simulink model "siso_4_channel_teleop_force"  (R2021a)
settings: Solver=VariableStepAuto  StartTime=0.0  StopTime=5  FixedStep=Ts  RelTol=1e-3
values from neighbouring files (symbols this model uses):
  A = pi/4    (= 0.785398163397)    [assignment2.m]
  Be = 100    [assignment2.m]
  Bh = 7    [assignment2.m]
  Bm = 100    [assignment2.m]
  Bs = 1000    [assignment2.m]
  Cmf = -0.67    [assignment2.m]
  Csf = -0.67    [assignment2.m]
  Dh = 500    [assignment2.m]
  Dm = 0    [assignment2.m]
  Ds = 0    [assignment2.m]
  Fc = 1    [assignment2.m]
  Flp = 5    [assignment2.m]
  Jh = 0.05    [assignment2.m]
  k_h = 8000    [assignment2.m]
  Ke = 200    [assignment2.m]
  Kh = 200    [assignment2.m]
  Km = 500    [assignment2.m]
  Ks = 80000    [assignment2.m]
  Mm = 0.5    [assignment2.m]
  Ms = 2    [assignment2.m]
  Ts = 0.001    [assignment2.m]
  xe = 1    [assignment2.m]
libraries: simulink x2
settings Model: Creator=fabio  LastModifiedBy=fabio

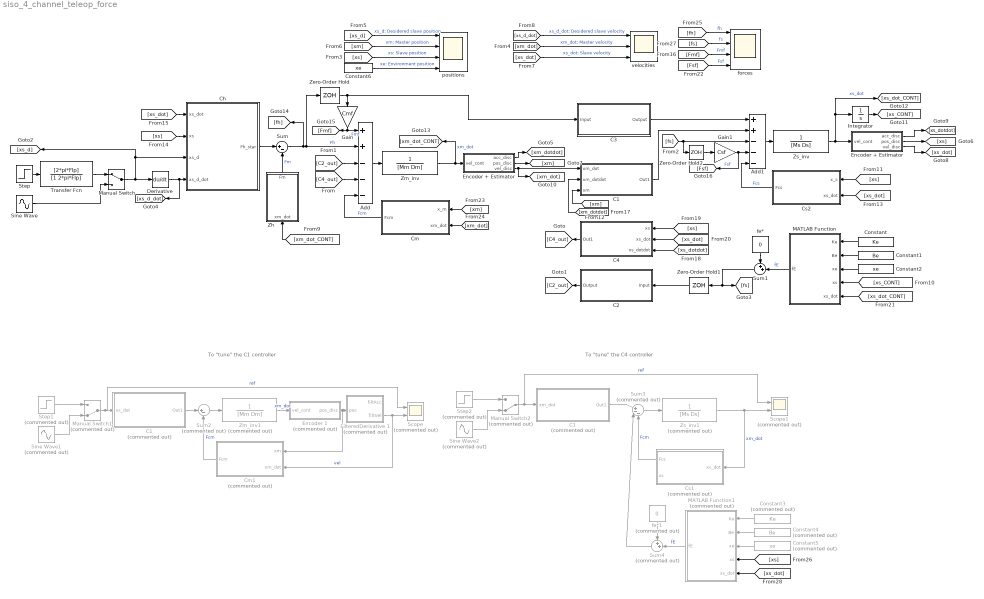
== system siso_4_channel_teleop_force ==
  note: To "tune" the C1 controller
  note: To "tune" the C4 controller
  Add : Sum  Inputs=++---
  Add1 : Sum  Inputs=++---
  C1 : Subsystem
  "C1 " : Subsystem  Commented=on
  "C1    " : Subsystem  Commented=on
  C2 : Subsystem
  C3 : Subsystem
  C4 : Subsystem
  Ch : Subsystem
  Cm : Subsystem
  Cm1 : Subsystem  Commented=on
  Constant : Constant  Value=Ke
  Constant1 : Constant  Value=Be
  Constant2 : Constant  Value=xe
  Constant3 : Constant  Commented=on  Value=Ke
  Constant4 : Constant  Commented=on  Value=Be
  Constant5 : Constant  Commented=on  Value=xe
  Constant6 : Constant  Value=xe
  Cs1 : Subsystem  Commented=on
  Cs2 : Subsystem
  Derivative : Derivative
  Encoder + Estimator : Subsystem
  "Encoder + Estimator " : Subsystem
  Encoder 1 : Subsystem  Commented=on
  FilteredDerivative 1 : Subsystem  Commented=on
  Gain : Gain  Gain=Cmf
  Gain1 : Gain  Gain=Csf
  Integrator : Integrator
  MATLAB Function : MATLAB Function  TreatAsAtomicUnit=on
  MATLAB Function1 : MATLAB Function  Commented=on  TreatAsAtomicUnit=on
  Manual Switch : ManualSwitch
  Manual Switch1 : ManualSwitch  Commented=on  CurrentSetting=0
  Manual Switch2 : ManualSwitch  Commented=on  CurrentSetting=0
  Scope : Scope  Commented=on  NumInputPorts=2
  Scope1 : Scope  Commented=on  NumInputPorts=2
  Sine Wave : Sin  Amplitude=A  Frequency=Fc*2*pi  SampleTime=0
  Sine Wave1 : Sin  Commented=on  Amplitude=A  Frequency=Fc  SampleTime=0
  Sine Wave2 : Sin  Commented=on  Amplitude=A  Frequency=Fc  SampleTime=0
  Step : Step  After=A  SampleTime=0
  Step1 : Step  Commented=on  SampleTime=0
  Step2 : Step  Commented=on  SampleTime=0
  Sum : Sum  Inputs=|+-
  Sum1 : Sum  Inputs=++|
  Sum2 : Sum  Commented=on  Inputs=|+-
  Sum3 : Sum  Commented=on  Inputs=|+--
  Sum4 : Sum  Commented=on  Inputs=++|
  Transfer Fcn : TransferFcn  Numerator=[2*pi*Flp]  Denominator=[1 2*pi*Flp]
  Zero-Order Hold : ZeroOrderHold  SampleTime=Ts
  Zero-Order Hold1 : ZeroOrderHold  SampleTime=Ts
  Zero-Order Hold2 : ZeroOrderHold  SampleTime=Ts
  Zh : Subsystem
  Zm_inv : TransferFcn  Numerator=[0 1]  Denominator=[Mm Dm]
  Zm_inv1 : TransferFcn  Commented=on  Numerator=[0 1]  Denominator=[Mm Dm]
  Zs_inv : TransferFcn  Numerator=[0 1]  Denominator=[Ms Ds]
  Zs_inv1 : TransferFcn  Commented=on  Numerator=[0 1]  Denominator=[Ms Ds]
  fe* : Constant  Value=0
  fe*1 : Constant  Commented=on  Value=0
  forces : Scope  NumInputPorts=4
  positions : Scope  NumInputPorts=4
  velocities : Scope  NumInputPorts=3
  wires:
  Zh/1(Fm) -> Sum/2  "Fm"
  Sum/1 -> Add/2, Zero-Order Hold/1, [fh]  "Fh"
  Add/1 -> Zm_inv/1
  Cm/1(Fcm) -> Add/5  "Fcm"
  Cs2/1(Fcs) -> Add1/5  "Fcs"
  Add1/1 -> Zs_inv/1
  Constant/1 -> MATLAB Function/1(Ke)
  Constant1/1 -> MATLAB Function/2(Be)
  Constant2/1 -> MATLAB Function/3(xe)
  [xs_CONT] -> MATLAB Function/4(xs)
  [xs_dot_CONT] -> MATLAB Function/5(xs_dot)
  MATLAB Function/1(fE) -> Sum1/2  "fE"
  C4/1(Out1) -> [C4_out]
  [C4_out] -> Add/4
  C3/1(Output) -> Add1/1
  [fs] -> Add1/3, Zero-Order Hold2/1
  C2/1(Output) -> [C2_out]
  Ch/1(Fh_star) -> Sum/1
  [C2_out] -> Add/3
  [xs_d] -> positions/1  "xs_d: Desidered slave position"
  [xm] -> positions/2  "xm: Master position"
  [xs] -> positions/3  "xs: Slave position"
  [xm_dot] -> velocities/2  "xm_dot: Master velocity"
  [xs_dot] -> velocities/3  "xs_dot: Slave velocity"
  [xs_d_dot] -> velocities/1  "xs_d_dot: Desidered slave velocity"
  [xs_dot] -> Ch/4(xs_dot)
  [xs] -> Ch/3(xs)
  Sine Wave/1 -> Manual Switch/2
  Derivative/1 -> [xs_d_dot], Ch/1(xs_d_dot)
  fe*/1 -> Sum1/1
  Sum2/1 -> Zm_inv1/1
  Cm1/1(Fcm) -> Sum2/2  "Fcm"
  "C1    "/1(Out1) -> Sum2/1
  Step1/1 -> Manual Switch1/1
  Sine Wave1/1 -> Manual Switch1/2
  Manual Switch1/1 -> Scope/1, "C1    "/1(xs_dot)  "ref"
  Manual Switch2/1 -> "C1 "/1(xm_dot), Scope1/1  "ref"
  Sine Wave2/1 -> Manual Switch2/2
  Step2/1 -> Manual Switch2/1
  "C1 "/1(Out1) -> Sum3/1
  Zs_inv1/1 -> Cs1/1(xs_dot), Scope1/2  "xm_dot"
  Sum3/1 -> Zs_inv1/1
  fe*1/1 -> Sum4/1
  [xs] -> MATLAB Function1/4(xs)
  MATLAB Function1/1(fE) -> Sum4/2  "fE"
  Constant3/1 -> MATLAB Function1/1(Ke)
  [xs_dot] -> MATLAB Function1/5(xs_dot)
  Constant4/1 -> MATLAB Function1/2(Be)
  Constant5/1 -> MATLAB Function1/3(xe)
  Cs1/1(Fcs) -> Sum3/3  "Fcm"
  Sum4/1 -> Sum3/2
  Step/1 -> Transfer Fcn/1
  Transfer Fcn/1 -> Manual Switch/1
  Zs_inv/1 -> [xs_dot_CONT], Integrator/1, "Encoder + Estimator "/1(vel_cont)  "xs_dot"
  Zm_inv/1 -> [xm_dot_CONT], Encoder + Estimator/1(vel_cont)  "xm_dot"
  "Encoder + Estimator "/3(vel_disc) -> [xs_dot]
  Zero-Order Hold1/1 -> C2/1(Input)
  Manual Switch/1 -> Ch/2(xs_d), [xs_d], Derivative/1
  "Encoder + Estimator "/1(acc_disc) -> [xs_dotdot]
  [xs] -> C4/1(xs)
  [xs_dotdot] -> C4/3(xs_dotdot)
  [xs_dot] -> C4/2(xs_dot)
  Integrator/1 -> [xs_CONT]
  [xs] -> Cs2/1(x_s)
  [xs_dot] -> Cs2/2(xs_dot)
  Zero-Order Hold/1 -> Gain/1, C3/1(Input)
  Encoder + Estimator/1(acc_disc) -> [xm_dotdot]
  [xm] -> C1/3(xm)
  [xm_dotdot] -> C1/2(xm_dotdot)
  Sum1/1 -> [fs], Zero-Order Hold1/1
  [xm] -> Cm/1(x_m)
  [xm_dot] -> Cm/2(xm_dot)
  Zm_inv1/1 -> Encoder 1/1(vel_cont)  "xm_dot"
  Encoder 1/1(pos_disc) -> Cm1/1(xm), FilteredDerivative 1/1(pos)
  FilteredDerivative 1/2(filtVel) -> Cm1/2(xm_dot), Scope/2  "vel"
  [xm_dot_CONT] -> Zh/1(xm_dot)
  C1/1(Out1) -> Add1/2
  Encoder + Estimator/3(vel_disc) -> C1/1(xm_dot), [xm_dot]
  Encoder + Estimator/2(pos_disc) -> [xm]
  "Encoder + Estimator "/2(pos_disc) -> [xs]
  Constant6/1 -> positions/4  "xe: Environment position"
  [fh] -> forces/1  "fh"
  [fs] -> forces/2  "fs"
  Gain/1 -> Add/1, [Fmf]  "Fmf"
  Gain1/1 -> [Fsf], Add1/4  "Fsf"
  Zero-Order Hold2/1 -> Gain1/1
  [Fmf] -> forces/3  "Fmf"
  [Fsf] -> forces/4  "Fsf"

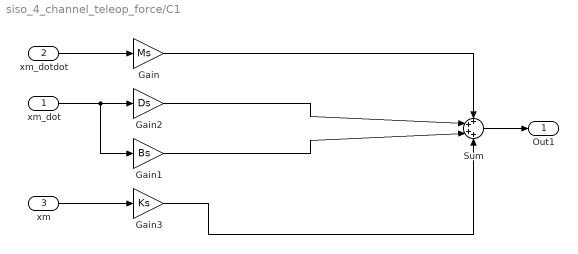
== system siso_4_channel_teleop_force/C1 ==
  xm_dot : Inport
  xm_dotdot : Inport  Port=2
  xm : Inport  Port=3
  Gain : Gain  Gain=Ms
  Gain1 : Gain  Gain=Bs
  Gain2 : Gain  Gain=Ds
  Gain3 : Gain  Gain=Ks
  Sum : Sum  Inputs=++++
  Out1 : Outport
  wires:
  Gain/1 -> Sum/1
  Gain2/1 -> Sum/2
  Gain1/1 -> Sum/3
  Gain3/1 -> Sum/4
  Sum/1 -> Out1/1
  xm/1 -> Gain3/1
  xm_dot/1 -> Gain1/1, Gain2/1
  xm_dotdot/1 -> Gain/1

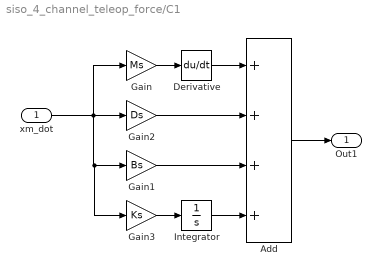
== system siso_4_channel_teleop_force/C1  ==
  xm_dot : Inport
  Add : Sum  Inputs=++++
  Derivative : Derivative
  Gain : Gain  Gain=Ms
  Gain1 : Gain  Gain=Bs
  Gain2 : Gain  Gain=Ds
  Gain3 : Gain  Gain=Ks
  Integrator : Integrator
  Out1 : Outport
  wires:
  Add/1 -> Out1/1
  Integrator/1 -> Add/4
  Gain3/1 -> Integrator/1
  Gain1/1 -> Add/3
  Gain2/1 -> Add/2
  Derivative/1 -> Add/1
  Gain/1 -> Derivative/1
  xm_dot/1 -> Gain2/1, Gain1/1, Gain3/1, Gain/1

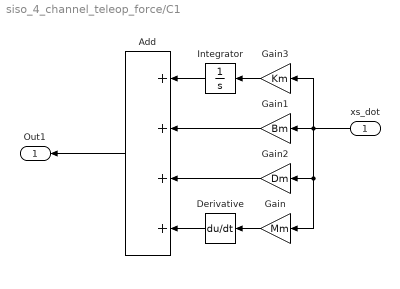
== system siso_4_channel_teleop_force/C1     ==
  xs_dot : Inport
  Add : Sum  Inputs=++++
  Derivative : Derivative
  Gain : Gain  Gain=Mm
  Gain1 : Gain  Gain=Bm
  Gain2 : Gain  Gain=Dm
  Gain3 : Gain  Gain=Km
  Integrator : Integrator
  Out1 : Outport
  wires:
  Add/1 -> Out1/1
  Integrator/1 -> Add/1
  Gain1/1 -> Add/2
  Gain2/1 -> Add/3
  Derivative/1 -> Add/4
  xs_dot/1 -> Gain1/1, Gain3/1, Gain2/1, Gain/1
  Gain/1 -> Derivative/1
  Gain3/1 -> Integrator/1

== system siso_4_channel_teleop_force/C2 ==
  Input : Inport
  Output : Outport
  wires:
  Input/1 -> Output/1

== system siso_4_channel_teleop_force/C3 ==
  Input : Inport
  Output : Outport
  wires:
  Input/1 -> Output/1

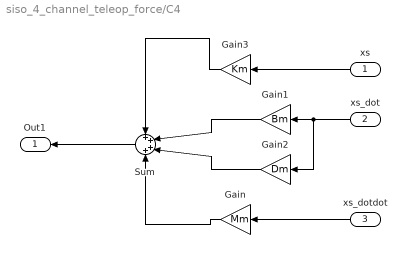
== system siso_4_channel_teleop_force/C4 ==
  xs : Inport
  xs_dot : Inport  Port=2
  xs_dotdot : Inport  Port=3
  Gain : Gain  Gain=Mm
  Gain1 : Gain  Gain=Bm
  Gain2 : Gain  Gain=Dm
  Gain3 : Gain  Gain=Km
  Sum : Sum  Inputs=++++
  Out1 : Outport
  wires:
  xs_dot/1 -> Gain2/1, Gain1/1
  Gain/1 -> Sum/4
  Gain2/1 -> Sum/3
  Gain1/1 -> Sum/2
  Gain3/1 -> Sum/1
  Sum/1 -> Out1/1
  xs_dotdot/1 -> Gain/1
  xs/1 -> Gain3/1

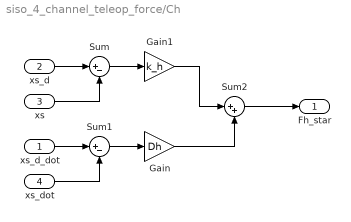
== system siso_4_channel_teleop_force/Ch ==
  xs_d_dot : Inport
  xs_d : Inport  Port=2
  xs : Inport  Port=3
  xs_dot : Inport  Port=4
  Gain : Gain  Gain=Dh
  Gain1 : Gain  Gain=k_h
  Sum : Sum  Inputs=|+-
  Sum1 : Sum  Inputs=|+-
  Sum2 : Sum  Inputs=|++
  Fh_star : Outport
  wires:
  Gain1/1 -> Sum2/1
  Sum2/1 -> Fh_star/1
  xs_d/1 -> Sum/1
  xs/1 -> Sum/2
  Sum/1 -> Gain1/1
  xs_dot/1 -> Sum1/2
  xs_d_dot/1 -> Sum1/1
  Sum1/1 -> Gain/1
  Gain/1 -> Sum2/2

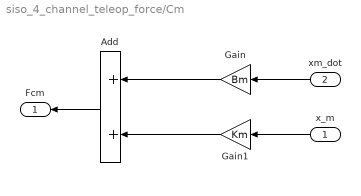
== system siso_4_channel_teleop_force/Cm ==
  x_m : Inport
  xm_dot : Inport  Port=2
  Add : Sum
  Gain : Gain  Gain=Bm
  Gain1 : Gain  Gain=Km
  Fcm : Outport
  wires:
  Gain1/1 -> Add/2
  xm_dot/1 -> Gain/1
  Gain/1 -> Add/1
  Add/1 -> Fcm/1
  x_m/1 -> Gain1/1

== system siso_4_channel_teleop_force/Cm1 ==
  xm : Inport
  xm_dot : Inport  Port=2
  Add : Sum
  Gain : Gain  Gain=Bm
  Gain1 : Gain  Gain=Km
  Fcm : Outport
  wires:
  Gain1/1 -> Add/2
  Add/1 -> Fcm/1
  Gain/1 -> Add/1
  xm_dot/1 -> Gain/1
  xm/1 -> Gain1/1

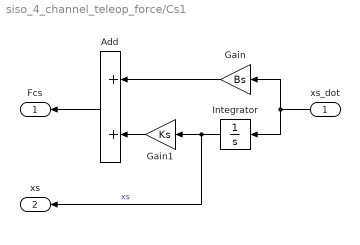
== system siso_4_channel_teleop_force/Cs1 ==
  xs_dot : Inport
  Add : Sum
  Gain : Gain  Gain=Bs
  Gain1 : Gain  Gain=Ks
  Integrator : Integrator
  Fcs : Outport
  xs : Outport  Port=2
  wires:
  Add/1 -> Fcs/1
  xs_dot/1 -> Integrator/1, Gain/1
  Gain/1 -> Add/1
  Integrator/1 -> xs/1, Gain1/1  "xs"
  Gain1/1 -> Add/2

== system siso_4_channel_teleop_force/Cs2 ==
  x_s : Inport
  xs_dot : Inport  Port=2
  Add : Sum
  Gain : Gain  Gain=Bs
  Gain1 : Gain  Gain=Ks
  Fcs : Outport
  wires:
  Add/1 -> Fcs/1
  xs_dot/1 -> Gain/1
  Gain/1 -> Add/1
  x_s/1 -> Gain1/1  "xs"
  Gain1/1 -> Add/2

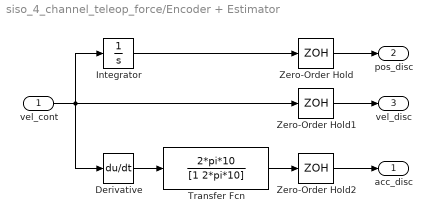
== system siso_4_channel_teleop_force/Encoder + Estimator ==
  vel_cont : Inport
  Derivative : Derivative
  Integrator : Integrator
  Transfer Fcn : TransferFcn  Numerator=2*pi*10  Denominator=[1 2*pi*10]
  Zero-Order Hold : ZeroOrderHold  SampleTime=Ts
  Zero-Order Hold1 : ZeroOrderHold  SampleTime=Ts
  Zero-Order Hold2 : ZeroOrderHold  SampleTime=Ts
  acc_disc : Outport
  pos_disc : Outport  Port=2
  vel_disc : Outport  Port=3
  wires:
  Zero-Order Hold/1 -> pos_disc/1
  vel_cont/1 -> Derivative/1, Integrator/1, Zero-Order Hold1/1
  Integrator/1 -> Zero-Order Hold/1
  Zero-Order Hold1/1 -> vel_disc/1
  Zero-Order Hold2/1 -> acc_disc/1
  Derivative/1 -> Transfer Fcn/1
  Transfer Fcn/1 -> Zero-Order Hold2/1

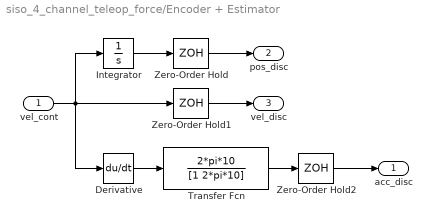
== system siso_4_channel_teleop_force/Encoder + Estimator  ==
  vel_cont : Inport
  Derivative : Derivative
  Integrator : Integrator
  Transfer Fcn : TransferFcn  Numerator=2*pi*10  Denominator=[1 2*pi*10]
  Zero-Order Hold : ZeroOrderHold  SampleTime=Ts
  Zero-Order Hold1 : ZeroOrderHold  SampleTime=Ts
  Zero-Order Hold2 : ZeroOrderHold  SampleTime=Ts
  acc_disc : Outport
  pos_disc : Outport  Port=2
  vel_disc : Outport  Port=3
  wires:
  Zero-Order Hold/1 -> pos_disc/1
  vel_cont/1 -> Derivative/1, Integrator/1, Zero-Order Hold1/1
  Integrator/1 -> Zero-Order Hold/1
  Zero-Order Hold1/1 -> vel_disc/1
  Zero-Order Hold2/1 -> acc_disc/1
  Derivative/1 -> Transfer Fcn/1
  Transfer Fcn/1 -> Zero-Order Hold2/1

== system siso_4_channel_teleop_force/Encoder 1 ==
  vel_cont : Inport
  Integrator1 : Integrator
  Zero-Order Hold : ZeroOrderHold  SampleTime=Ts
  pos_disc : Outport
  wires:
  Zero-Order Hold/1 -> pos_disc/1
  vel_cont/1 -> Integrator1/1
  Integrator1/1 -> Zero-Order Hold/1

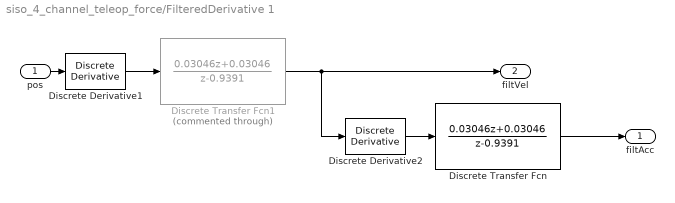
== system siso_4_channel_teleop_force/FilteredDerivative 1 ==
  pos : Inport
  Discrete Transfer Fcn : DiscreteTransferFcn  Numerator=[0.03046 0.03046]  Denominator=[1 -0.9391]
  Discrete Transfer Fcn1 : DiscreteTransferFcn  Commented=through  Numerator=[0.03046 0.03046]  Denominator=[1 -0.9391]
  Discrete Derivative1 : simulink/Discrete/Discrete Derivative  gainval=1.0  ICPrevScaledInput=0.0  OutMin=[]  OutMax=[]  OutDataType=fixdt(1, 16)  OutScaling=2^-10  DoSatur=off
  Discrete Derivative2 : simulink/Discrete/Discrete Derivative  gainval=1.0  ICPrevScaledInput=0.0  OutMin=[]  OutMax=[]  OutDataType=fixdt(1, 16)  OutScaling=2^-10  DoSatur=off
  filtAcc : Outport
  filtVel : Outport  Port=2
  wires:
  pos/1 -> Discrete Derivative1/1
  Discrete Derivative1/1 -> Discrete Transfer Fcn1/1
  Discrete Derivative2/1 -> Discrete Transfer Fcn/1
  Discrete Transfer Fcn/1 -> filtAcc/1
  Discrete Transfer Fcn1/1 -> Discrete Derivative2/1, filtVel/1

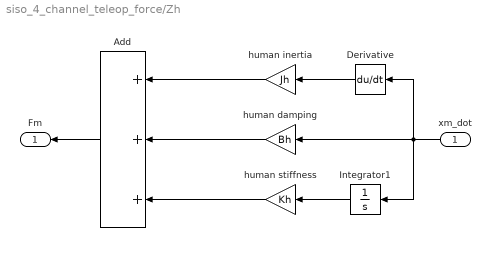
== system siso_4_channel_teleop_force/Zh ==
  xm_dot : Inport
  Add : Sum  Inputs=+++
  Derivative : Derivative
  Integrator1 : Integrator
  human damping : Gain  Gain=Bh
  human inertia : Gain  Gain=Jh
  human stiffness : Gain  Gain=Kh
  Fm : Outport
  wires:
  Add/1 -> Fm/1
  human inertia/1 -> Add/1
  human stiffness/1 -> Add/3
  human damping/1 -> Add/2
  xm_dot/1 -> Integrator1/1, Derivative/1, human damping/1
  Integrator1/1 -> human stiffness/1
  Derivative/1 -> human inertia/1

== matlab function siso_4_channel_teleop_force/MATLAB Function1 ==
  data: Ke input; fE output; Be input; xe input; xs input; xs_dot input
function fE = environment(Ke, Be, xe, xs, xs_dot)
    if xs > xe
        fE = Ke*(xs - xe) + Be*xs_dot;
    else
        fE = 0;
    end
end

== matlab function siso_4_channel_teleop_force/MATLAB Function ==
  data: Ke input; fE output; Be input; xe input; xs input; xs_dot input
function fE = environment(Ke, Be, xe, xs, xs_dot)
    if xs > xe
        fE = Ke*(xs - xe) + Be*xs_dot;
    else
        fE = 0;
    end
end
